simulink model "WAOPSQ"  (R2016a)
settings: Solver=VariableStepAuto  StartTime=0.0  StopTime=100  RelTol=1e-3
undefined symbols (not defined in the file or in its folder): m, n
libraries: commrandsrc3 x1, dspstat3 x1
settings Model: Creator=demo  LastModifiedBy=demo

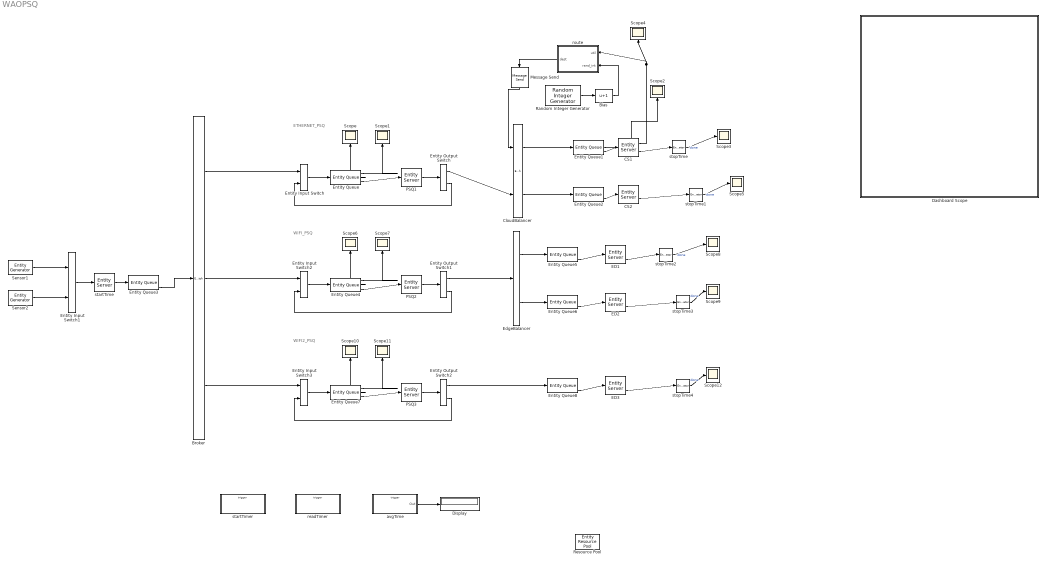
== system WAOPSQ ==
  note: ETHERNET_PSQ
  note: WIFI_PSQ
  note: WIFI2_PSQ
  Bias : Bias  Bias=1
  Broker : EntityOutputSwitch  InputPortMessageModes=m  OutputPortMessageModes=m,m,m  NumberOutputPorts=3  SwitchingCriterion=Equiprobable  SwitchAttributeName=dest
      settings: OutputPortMap=o0,o1,o2
  CS1 : EntityServer  InputPortMessageModes=m  OutputPortMessageModes=n,m  Capacity=1  ServiceTimeValue=2  ServiceTimeAttributeName=timeSlice  WriteResidualTimeToAttribute=on  ResidualTimeAttributeName=PreemptionPriority  Utilization=on
      settings: OutputPortMap=o5,o9
  CS2 : EntityServer  InputPortMessageModes=m  OutputPortMessageModes=n,m  Capacity=1  ServiceTimeValue=2  ServiceTimeAttributeName=timeSlice  WriteResidualTimeToAttribute=on  ResidualTimeAttributeName=PreemptionPriority  Utilization=on
      settings: OutputPortMap=o5,o9
  CloudBalancer : EntityOutputSwitch  InputPortMessageModes=m,m  OutputPortMessageModes=m,m  SwitchingCriterion=From control port  SwitchAttributeName=dest
      settings: InputPortMap=u0,u1
  Dashboard Scope : Subsystem  DialogController=hmiCreateDDGDialog  IsWebBlock=on  mask(MWDashboardBlock){webBlockId=93fdf2d6-6c09-4820-8f1f-cc3ef1f549fc, webBlockType=sdiscope, ShowInitialText=on, HMISrcModelName=WAOPSQ}
      mask prompts: webBlockId "WebBlock Id"; webBlockType "WebBlock Type"; HMISrcModelName "Source Model"
      mask Help: helpview([docroot '/mapfiles/simulink.map'], 'hmi_scope')
      mask Display:
      | if strcmp(get_param(bdroot(gcb),'BlockDiagramType'), 'library')
      |     image([(matlabroot) '/toolbox/simulink/hmi/icons/DashboardScope.png']);
      | end
  Display : Display
  ED1 : EntityServer  InputPortMessageModes=m  OutputPortMessageModes=n,m  Capacity=1  ServiceTimeValue=2  ServiceTimeAttributeName=timeSlice  WriteResidualTimeToAttribute=on  ResidualTimeAttributeName=PreemptionPriority  Utilization=on
      settings: OutputPortMap=o5,o9
  ED2 : EntityServer  InputPortMessageModes=m  OutputPortMessageModes=n,m  Capacity=1  ServiceTimeValue=2  ServiceTimeAttributeName=timeSlice  WriteResidualTimeToAttribute=on  ResidualTimeAttributeName=PreemptionPriority  Utilization=on
      settings: OutputPortMap=o5,o9
  ED3 : EntityServer  InputPortMessageModes=m  OutputPortMessageModes=n,m  Capacity=1  ServiceTimeValue=2  ServiceTimeAttributeName=timeSlice  WriteResidualTimeToAttribute=on  ResidualTimeAttributeName=PreemptionPriority  Utilization=on
      settings: OutputPortMap=o5,o9
  EdgeBalancer : EntityOutputSwitch  InputPortMessageModes=m  OutputPortMessageModes=m,m  SwitchingCriterion=Round robin  SwitchAttributeName=dest
  Entity Input Switch{,1..3} (4 alike) : EntityInputSwitch  InputPortMessageModes=m,m  OutputPortMessageModes=m
  Entity Output Switch : EntityOutputSwitch  InputPortMessageModes=m  OutputPortMessageModes=m,m  SwitchingCriterion=From attribute  SwitchAttributeName=dest
  Entity Output Switch1 : EntityOutputSwitch  InputPortMessageModes=m  OutputPortMessageModes=m,m  SwitchingCriterion=From attribute  SwitchAttributeName=dest
  Entity Output Switch2 : EntityOutputSwitch  InputPortMessageModes=m  OutputPortMessageModes=m,m  SwitchingCriterion=From attribute  SwitchAttributeName=dest
  Entity Queue{,1..8} (9 alike) : EntityQueue  InputPortMessageModes=m  OutputPortMessageModes=n,n,m  NumberEntitiesDeparted=on  NumberEntitiesInBlock=on
      settings: OutputPortMap=o0,o1,o5
  Message Send : MessageSend  OutputPortMessageModes=m
      settings: InputPortMap=u1
  PSQ1 : EntityServer  InputPortMessageModes=m  OutputPortMessageModes=m  Capacity=1  ServiceTimeSource=Attribute  ServiceTimeValue=.2  ServiceTimeAttributeName=timeSlice  ServiceCompleteAction=|  WriteResidualTimeToAttribute=on  ResidualTimeAttributeName=PreemptionPriority
      | entity.ServiceTime = entity.ServiceTime - entity.timeSlice
      | 
      | if(entity.ServiceTime < abs(eps))
      |     entity.dest = 1
      | else
      |     entity.dest = 2
  PSQ2 : EntityServer  InputPortMessageModes=m  OutputPortMessageModes=m  Capacity=1  ServiceTimeSource=Attribute  ServiceTimeValue=.2  ServiceTimeAttributeName=timeSlice  ServiceCompleteAction=|  WriteResidualTimeToAttribute=on  ResidualTimeAttributeName=PreemptionPriority
      | entity.ServiceTime = entity.ServiceTime - entity.timeSlice
      | 
      | if(entity.ServiceTime < abs(eps))
      |     entity.dest = 1
      | else
      |     entity.dest = 2
  PSQ3 : EntityServer  InputPortMessageModes=m  OutputPortMessageModes=m  Capacity=1  ServiceTimeSource=Attribute  ServiceTimeValue=.2  ServiceTimeAttributeName=timeSlice  ServiceCompleteAction=|  WriteResidualTimeToAttribute=on  ResidualTimeAttributeName=PreemptionPriority
      | entity.ServiceTime = entity.ServiceTime - entity.timeSlice
      | 
      | if(entity.ServiceTime < abs(eps))
      |     entity.dest = 1
      | else
      |     entity.dest = 2
  Random Integer Generator : commrandsrc3/Random Integer Generator  SetSize=2  SeedSource=Auto  Seed=0  SampleTime=1  SamplesPerFrame=1  OutputDataType=double  SimulateUsing=Interpreted execution
  Resource Pool : EntityResourcePool
  Scope{,1..12} (13 alike) : Scope
  Sensor1 : EntityGenerator  OutputPortMessageModes=m  Period=2  AttributeName=ServiceTime|timer|dest|timeSlice  AttributeInitialValue=2|0|1|.2  EntityType=Structured  EntityTypeName=Entity
  Sensor2 : EntityGenerator  OutputPortMessageModes=m  Period=200  AttributeName=ServiceTime|timer|dest|timeSlice  AttributeInitialValue=2|0|1|.2  EntityType=Structured  EntityTypeName=Entity
  avgTime : Subsystem  TreatAsAtomicUnit=on
  readTimer : Subsystem  TreatAsAtomicUnit=on
  route : Stateflow chart  TreatAsAtomicUnit=on
  startTime : EntityServer  InputPortMessageModes=m  OutputPortMessageModes=m  Capacity=1  ServiceTimeValue=0  ServiceTimeAttributeName=PreemptionPriority  EntryAction=entity.timer = startTimer();  WriteResidualTimeToAttribute=on  ResidualTimeAttributeName=PreemptionPriority
  startTimer : Subsystem  TreatAsAtomicUnit=on
  stopTime : EntityTerminator  InputPortMessageModes=m  EntryAction=|  NumberEntitiesArrived=on
      | % Read timer
      | elapsedTime = readTimer(entity.timer);
      | 
      | % Compute average
      | avgTime(elapsedTime);
      settings: OutputPortMap=o0
  stopTime1 : EntityTerminator  InputPortMessageModes=m  EntryAction=|  NumberEntitiesArrived=on
      | % Read timer
      | elapsedTime = readTimer(entity.timer);
      | 
      | % Compute average
      | avgTime(elapsedTime);
      settings: OutputPortMap=o0
  stopTime2 : EntityTerminator  InputPortMessageModes=m  EntryAction=|  NumberEntitiesArrived=on
      | % Read timer
      | elapsedTime = readTimer(entity.timer);
      | 
      | % Compute average
      | avgTime(elapsedTime);
      settings: OutputPortMap=o0
  stopTime3 : EntityTerminator  InputPortMessageModes=m  EntryAction=|  NumberEntitiesArrived=on
      | % Read timer
      | elapsedTime = readTimer(entity.timer);
      | 
      | % Compute average
      | avgTime(elapsedTime);
      settings: OutputPortMap=o0
  stopTime4 : EntityTerminator  InputPortMessageModes=m  EntryAction=|  NumberEntitiesArrived=on
      | % Read timer
      | elapsedTime = readTimer(entity.timer);
      | 
      | % Compute average
      | avgTime(elapsedTime);
      settings: OutputPortMap=o0
  wires:
  stopTime/1 -> Scope3/1  "done"
  avgTime/1(Out) -> Display/1
  Entity Queue/1 -> Scope1/1
  Entity Queue/3 -> PSQ1/1
  Entity Input Switch/1 -> Entity Queue/1
  Entity Queue/2 -> Scope/1
  Entity Output Switch/2 -> Entity Input Switch/2
  PSQ1/1 -> Entity Output Switch/1
  Sensor1/1 -> Entity Input Switch1/1
  Sensor2/1 -> Entity Input Switch1/2
  Entity Input Switch1/1 -> startTime/1
  Entity Output Switch/1 -> CloudBalancer/2
  Broker/1 -> Entity Input Switch/1
  CloudBalancer/1 -> Entity Queue1/1
  Entity Queue1/3 -> CS1/1
  CS1/2 -> stopTime/1
  CS1/1 -> Scope4/1, route/1(util)
  Message Send/1 -> CloudBalancer/1
  Random Integer Generator/1 -> Bias/1
  Bias/1 -> route/2(rand_int)
  Entity Queue1/2 -> Scope2/1
  route/1(dest) -> Message Send/1
  CloudBalancer/2 -> Entity Queue2/1
  Entity Queue2/3 -> CS2/1
  stopTime1/1 -> Scope5/1  "done"
  CS2/2 -> stopTime1/1
  startTime/1 -> Entity Queue3/1
  Entity Queue3/3 -> Broker/1
  Entity Queue4/1 -> Scope7/1
  Entity Queue4/3 -> PSQ2/1
  Entity Input Switch2/1 -> Entity Queue4/1
  Entity Queue4/2 -> Scope6/1
  Entity Output Switch1/2 -> Entity Input Switch2/2
  PSQ2/1 -> Entity Output Switch1/1
  Entity Output Switch1/1 -> EdgeBalancer/1
  Broker/2 -> Entity Input Switch2/1
  EdgeBalancer/1 -> Entity Queue5/1
  Entity Queue5/3 -> ED1/1
  EdgeBalancer/2 -> Entity Queue6/1
  Entity Queue6/3 -> ED2/1
  stopTime2/1 -> Scope8/1  "done"
  ED1/2 -> stopTime2/1
  stopTime3/1 -> Scope9/1  "done"
  ED2/2 -> stopTime3/1
  Entity Queue7/1 -> Scope11/1
  Entity Queue7/3 -> PSQ3/1
  Entity Input Switch3/1 -> Entity Queue7/1
  Entity Queue7/2 -> Scope10/1
  Entity Output Switch2/2 -> Entity Input Switch3/2
  PSQ3/1 -> Entity Output Switch2/1
  Broker/3 -> Entity Input Switch3/1
  Entity Queue8/3 -> ED3/1
  stopTime4/1 -> Scope12/1  "done"
  ED3/2 -> stopTime4/1
  Entity Output Switch2/1 -> Entity Queue8/1

== system WAOPSQ/Dashboard Scope ==

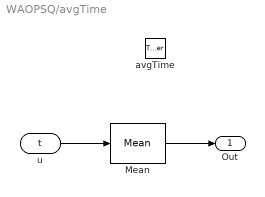
== system WAOPSQ/avgTime ==
  avgTime : TriggerPort  TriggerType=function-call  IsSimulinkFunction=on  FunctionName=avgTime  VariantControl=Variant
  Mean : dspstat3/Mean  run=off  reset_popup=None  InputProcessing=Columns as channels (frame based)  directionMode=Each column  dimension=1  roiEnable=off  roiType=Rectangles  roiPortion=Entire ROI  roiOutput=Individual statistics for each ROI  roiFlag=off  outputDataTypeStr=Inherit: Same as accumulator  outputLastDataTypeStr=Inherit: Same as accumulator  outputMin=[]  outputMax=[]  roundingMode=Floor  overflowMode=off
  u : ArgIn  DisableCoverage=on  ArgumentName=t
  Out : Outport
  wires:
  Mean/1 -> Out/1
  u/1 -> Mean/1

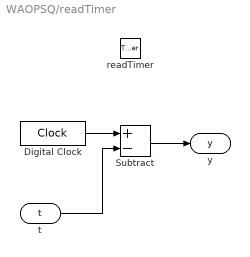
== system WAOPSQ/readTimer ==
  readTimer : TriggerPort  TriggerType=function-call  IsSimulinkFunction=on  FunctionName=readTimer  VariantControl=Variant
  Digital Clock : DigitalClock  SampleTime=-1
  Subtract : Sum  Inputs=+-
  t : ArgIn  DisableCoverage=on  ArgumentName=t
  y : ArgOut  DisableCoverage=on  ArgumentName=y
  wires:
  Digital Clock/1 -> Subtract/1
  Subtract/1 -> y/1
  t/1 -> Subtract/2

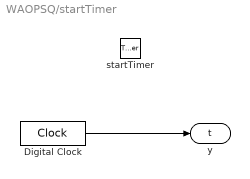
== system WAOPSQ/startTimer ==
  startTimer : TriggerPort  TriggerType=function-call  IsSimulinkFunction=on  FunctionName=startTimer  VariantControl=Variant
  Digital Clock : DigitalClock  SampleTime=-1
  y : ArgOut  DisableCoverage=on  ArgumentName=t
  wires:
  Digital Clock/1 -> y/1

== stateflow chart WAOPSQ/route ==
  state Route1
    en: dest = 1;
  state Route2
    en: dest = rand_int
    du: dest = rand_int
  (default) -> Route1
  Route2 -> Route1 : [util<.4]
  Route1 -> Route2 : [util>.7]
  data: dest output; x local; util input; rand_int input
